simulink model "CnvLead_Trq2Q"  (R2016b)
settings: configuration reference "CodeGenConfigSet" (kept outside this file)
values from neighbouring files (symbols this model uses):
  CnvLead_facRmpVal_CUR = Calibration.Parameter    [init_CnvLead_Trq2Q.m]    (also in init_CnvLead_Trq2Q_SIL.m = Simulink.Parameter)
  CnvLead_facRmpVal_CURX = Calibration.Parameter    [init_CnvLead_Trq2Q.m]    (also in init_CnvLead_Trq2Q_SIL.m = Simulink.Parameter)
  INJ_MASS_ZERO = fi(0,FuelMass_mg_hub)    [init_CnvLead_Trq2Q.m]    (also in init_CnvLead_Trq2Q_SIL.m)
  PhyMod_trq2qBas_MAP = Calibration.Parameter    [init_CnvLead_Trq2Q.m]    (also in init_CnvLead_Trq2Q_SIL.m = Simulink.Parameter)
  PhyMod_trq2qBas_MAPX = Calibration.Parameter    [init_CnvLead_Trq2Q.m]    (also in init_CnvLead_Trq2Q_SIL.m = Simulink.Parameter)
  PhyMod_trq2qBas_MAPY = Calibration.Parameter    [init_CnvLead_Trq2Q.m]    (also in init_CnvLead_Trq2Q_SIL.m = Simulink.Parameter)
libraries: simulink x2
settings Model: Creator=Colin  LastModifiedBy=zhoutinglin
settings ConfigSetRef: SourceLocation=Base Workspace

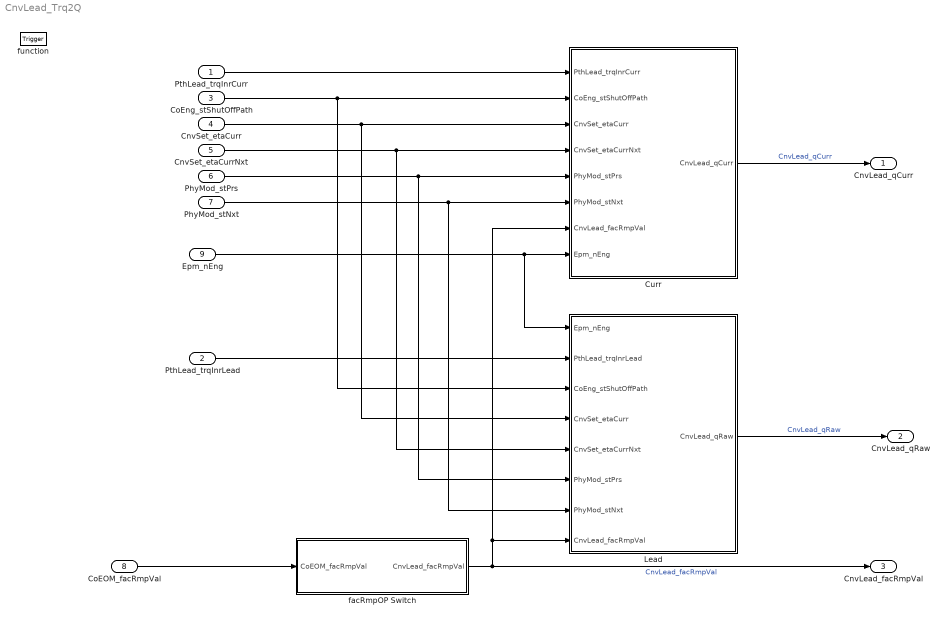
== system CnvLead_Trq2Q ==
  PthLead_trqInrCurr : Inport  Tag=Nm  Description=Actual percent engine torque  OutMin=-3000  OutMax=3000  OutDataTypeStr=Trq_Nm
  PthLead_trqInrLead : Inport  Tag=Nm  Description=Inner torque lead value  Port=2  OutMin=-3000  OutMax=3000  OutDataTypeStr=Trq_Nm
  CoEng_stShutOffPath : Inport  Description=Active shut-off paths resulting from active reversible,irreversible and afterrun shut-off paths  Port=3  OutMin=0  OutMax=65535  OutDataTypeStr=State_uint16
  CnvSet_etaCurr : Inport  Tag=Nm/(mg/hub)  Description=Current conversion efficiency  Port=4  OutMin=-255  OutMax=255  OutDataTypeStr=TrqEta_Nm_mg_hub
  CnvSet_etaCurrNxt : Inport  Tag=Nm/(mg/hub)  Description=conversion efficiency for next operation mode  Port=5  OutMin=-255  OutMax=255  OutDataTypeStr=TrqEta_Nm_mg_hub
  PhyMod_stPrs : Inport  Description=Current operating mode for the torque structure  Port=6  OutMin=0  OutMax=255  OutDataTypeStr=State_uint8
  PhyMod_stNxt : Inport  Description=Next operating mode for the torque structure  Port=7  OutMin=0  OutMax=255  OutDataTypeStr=State_uint8
  CoEOM_facRmpVal : Inport  Description=Central ramp value for operation mode change  Port=8  OutMin=-31  OutMax=31  OutDataTypeStr=Factor
  Epm_nEng : Inport  Tag=rpm  Description=Engine speed  Port=9  OutMin=0  OutMax=6000  OutDataTypeStr=EngSpeed_rpm
  function : TriggerPort  TriggerType=function-call  VariantControl=Variant
  Curr : Subsystem
  Lead : Subsystem
  facRmpOP Switch : Subsystem
  CnvLead_qCurr : Outport  Tag=mg/hub  Description=Injection quantity current path  OutMin=-319  OutMax=319  OutDataTypeStr=FuelMass_mg_hub
  CnvLead_qRaw : Outport  Tag=mg/hub  Description=Injection quantity raw path  Port=2  OutMin=-319  OutMax=319  OutDataTypeStr=FuelMass_mg_hub
  CnvLead_facRmpVal : Outport  Description=ramp factor  Port=3  OutMin=-31  OutMax=31  OutDataTypeStr=Factor
  wires:
  CoEOM_facRmpVal/1 -> facRmpOP Switch/1(CoEOM_facRmpVal)
  facRmpOP Switch/1(CnvLead_facRmpVal) -> Curr/7(CnvLead_facRmpVal), Lead/8(CnvLead_facRmpVal), CnvLead_facRmpVal/1  "CnvLead_facRmpVal"
  PthLead_trqInrCurr/1 -> Curr/1(PthLead_trqInrCurr)
  CoEng_stShutOffPath/1 -> Lead/3(CoEng_stShutOffPath), Curr/2(CoEng_stShutOffPath)
  CnvSet_etaCurr/1 -> Lead/4(CnvSet_etaCurr), Curr/3(CnvSet_etaCurr)
  CnvSet_etaCurrNxt/1 -> Lead/5(CnvSet_etaCurrNxt), Curr/4(CnvSet_etaCurrNxt)
  PhyMod_stPrs/1 -> Lead/6(PhyMod_stPrs), Curr/5(PhyMod_stPrs)
  PhyMod_stNxt/1 -> Lead/7(PhyMod_stNxt), Curr/6(PhyMod_stNxt)
  PthLead_trqInrLead/1 -> Lead/2(PthLead_trqInrLead)
  Curr/1(CnvLead_qCurr) -> CnvLead_qCurr/1  "CnvLead_qCurr"
  Lead/1(CnvLead_qRaw) -> CnvLead_qRaw/1  "CnvLead_qRaw"
  Epm_nEng/1 -> Lead/1(Epm_nEng), Curr/8(Epm_nEng)

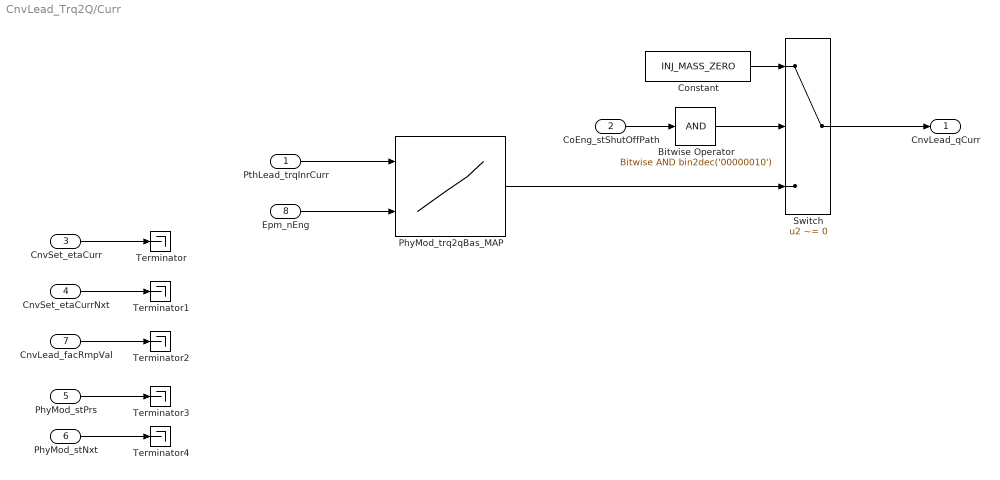
== system CnvLead_Trq2Q/Curr ==
  PthLead_trqInrCurr : Inport
  CoEng_stShutOffPath : Inport  Port=2
  CnvSet_etaCurr : Inport  Port=3
  CnvSet_etaCurrNxt : Inport  Port=4
  PhyMod_stPrs : Inport  Port=5
  PhyMod_stNxt : Inport  Port=6
  CnvLead_facRmpVal : Inport  Port=7
  Epm_nEng : Inport  Port=8
  Bitwise Operator : simulink/Logic and Bit Operations/Bitwise Operator  logicop=AND  UseBitMask=on  BitMask=bin2dec('00000010')  BitMaskRealWorld=Stored Integer
  Constant : Constant  Value=INJ_MASS_ZERO  OutDataTypeStr=FuelMass_mg_hub
  PhyMod_trq2qBas_MAP : Lookup_n-D  BreakpointsForDimension1=PhyMod_trq2qBas_MAPY  BreakpointsForDimension2=PhyMod_trq2qBas_MAPX  Table=PhyMod_trq2qBas_MAP  ExtrapMethod=Clip  InternalRulePriority=Speed  OutDataTypeStr=FuelMass_mg_hub  RndMeth=Simplest
  Switch : Switch  Criteria=u2 ~= 0  InputSameDT=on
  Terminator{,1..4} (5 alike) : Terminator
  CnvLead_qCurr : Outport
  wires:
  PhyMod_stPrs/1 -> Terminator3/1
  PhyMod_stNxt/1 -> Terminator4/1
  PhyMod_trq2qBas_MAP/1 -> Switch/3
  CoEng_stShutOffPath/1 -> Bitwise Operator/1
  Bitwise Operator/1 -> Switch/2
  Switch/1 -> CnvLead_qCurr/1
  Constant/1 -> Switch/1
  Epm_nEng/1 -> PhyMod_trq2qBas_MAP/2
  PthLead_trqInrCurr/1 -> PhyMod_trq2qBas_MAP/1
  CnvSet_etaCurr/1 -> Terminator/1
  CnvSet_etaCurrNxt/1 -> Terminator1/1
  CnvLead_facRmpVal/1 -> Terminator2/1

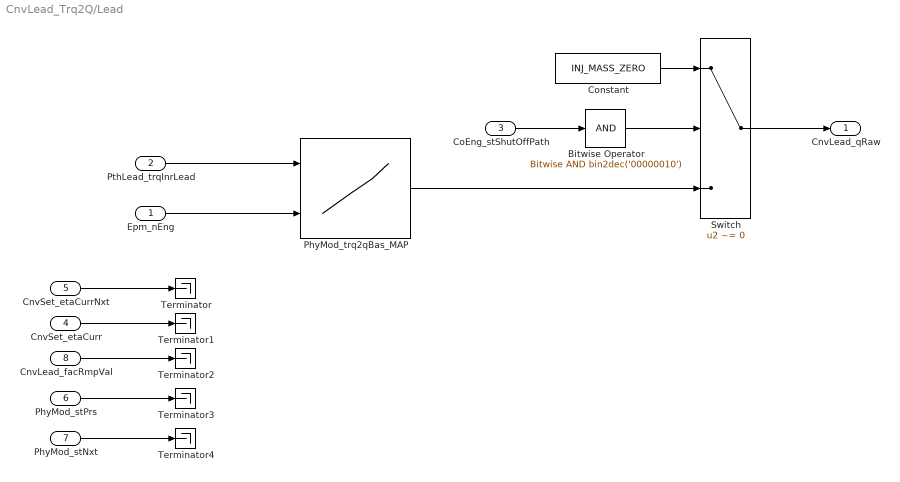
== system CnvLead_Trq2Q/Lead ==
  Epm_nEng : Inport
  PthLead_trqInrLead : Inport  Port=2
  CoEng_stShutOffPath : Inport  Port=3
  CnvSet_etaCurr : Inport  Port=4
  CnvSet_etaCurrNxt : Inport  Port=5
  PhyMod_stPrs : Inport  Port=6
  PhyMod_stNxt : Inport  Port=7
  CnvLead_facRmpVal : Inport  Port=8
  Bitwise Operator : simulink/Logic and Bit Operations/Bitwise Operator  logicop=AND  UseBitMask=on  BitMask=bin2dec('00000010')  BitMaskRealWorld=Stored Integer
  Constant : Constant  Value=INJ_MASS_ZERO  OutDataTypeStr=FuelMass_mg_hub
  PhyMod_trq2qBas_MAP : Lookup_n-D  BreakpointsForDimension1=PhyMod_trq2qBas_MAPY  BreakpointsForDimension2=PhyMod_trq2qBas_MAPX  Table=PhyMod_trq2qBas_MAP  ExtrapMethod=Clip  InternalRulePriority=Speed  OutDataTypeStr=FuelMass_mg_hub  RndMeth=Simplest
  Switch : Switch  Criteria=u2 ~= 0
  Terminator{,1..4} (5 alike) : Terminator
  CnvLead_qRaw : Outport
  wires:
  PhyMod_trq2qBas_MAP/1 -> Switch/3
  CoEng_stShutOffPath/1 -> Bitwise Operator/1
  Bitwise Operator/1 -> Switch/2
  Switch/1 -> CnvLead_qRaw/1
  Constant/1 -> Switch/1
  CnvSet_etaCurrNxt/1 -> Terminator/1
  CnvSet_etaCurr/1 -> Terminator1/1
  CnvLead_facRmpVal/1 -> Terminator2/1
  PhyMod_stPrs/1 -> Terminator3/1
  PhyMod_stNxt/1 -> Terminator4/1
  Epm_nEng/1 -> PhyMod_trq2qBas_MAP/2
  PthLead_trqInrLead/1 -> PhyMod_trq2qBas_MAP/1

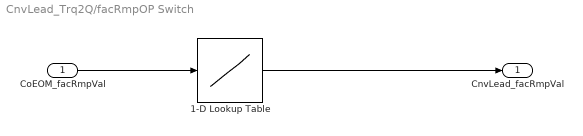
== system CnvLead_Trq2Q/facRmpOP Switch ==
  CoEOM_facRmpVal : Inport
  1-D Lookup Table : Lookup_n-D  NumberOfTableDimensions=1  BreakpointsForDimension1=CnvLead_facRmpVal_CURX  Table=CnvLead_facRmpVal_CUR  ExtrapMethod=Clip  InternalRulePriority=Speed  OutDataTypeStr=Inherit: Inherit via back propagation  RndMeth=Simplest  InputSameDT=on
  CnvLead_facRmpVal : Outport
  wires:
  CoEOM_facRmpVal/1 -> 1-D Lookup Table/1
  1-D Lookup Table/1 -> CnvLead_facRmpVal/1
